simulink model "labFinal_8.slx"  (R2018b)
settings: Solver=FixedStepDiscrete  StartTime=0.0  StopTime=10.0  FixedStep=1  RelTol=1e-3
libraries: hdlsllib x112, simulink_extras x8
(part 2 of 4)

== system labFinal_8.slx/8-Bit_Processor/8-bit Multiply/2^27 ==
  A : Inport
  B : Inport  Port=2
  Cin : Inport  Port=3
  Half_Adder : Subsystem
  Half_Adder1 : Subsystem
  Logical Operator : Logic  Operator=OR  AllPortsSameDT=off  OutDataTypeStr=boolean
  C : Outport
  S : Outport  Port=2
  wires:
  Half_Adder1/1(Sum) -> S/1
  Cin/1 -> Half_Adder1/2(y)
  Logical Operator/1 -> C/1
  Half_Adder1/2(Carry) -> Logical Operator/1
  A/1 -> Half_Adder/1(x)
  B/1 -> Half_Adder/2(y)
  Half_Adder/2(Carry) -> Logical Operator/2
  Half_Adder/1(Sum) -> Half_Adder1/1(x)

== system labFinal_8.slx/8-Bit_Processor/8-bit Multiply/2^28 ==
  A : Inport
  B : Inport  Port=2
  Cin : Inport  Port=3
  Half_Adder : Subsystem
  Half_Adder1 : Subsystem
  Logical Operator : Logic  Operator=OR  AllPortsSameDT=off  OutDataTypeStr=boolean
  C : Outport
  S : Outport  Port=2
  wires:
  Half_Adder1/1(Sum) -> S/1
  Cin/1 -> Half_Adder1/2(y)
  Logical Operator/1 -> C/1
  Half_Adder1/2(Carry) -> Logical Operator/1
  A/1 -> Half_Adder/1(x)
  B/1 -> Half_Adder/2(y)
  Half_Adder/2(Carry) -> Logical Operator/2
  Half_Adder/1(Sum) -> Half_Adder1/1(x)

== system labFinal_8.slx/8-Bit_Processor/8-bit Multiply/2^29 ==
  A : Inport
  B : Inport  Port=2
  Cin : Inport  Port=3
  Half_Adder : Subsystem
  Half_Adder1 : Subsystem
  Logical Operator : Logic  Operator=OR  AllPortsSameDT=off  OutDataTypeStr=boolean
  C : Outport
  S : Outport  Port=2
  wires:
  Half_Adder1/1(Sum) -> S/1
  Cin/1 -> Half_Adder1/2(y)
  Logical Operator/1 -> C/1
  Half_Adder1/2(Carry) -> Logical Operator/1
  A/1 -> Half_Adder/1(x)
  B/1 -> Half_Adder/2(y)
  Half_Adder/2(Carry) -> Logical Operator/2
  Half_Adder/1(Sum) -> Half_Adder1/1(x)

== system labFinal_8.slx/8-Bit_Processor/8-bit Multiply/2^3 ==
  A : Inport
  B : Inport  Port=2
  Cin : Inport  Port=3
  Half_Adder : Subsystem
  Half_Adder1 : Subsystem
  Logical Operator : Logic  Operator=OR  AllPortsSameDT=off  OutDataTypeStr=boolean
  C : Outport
  S : Outport  Port=2
  wires:
  Half_Adder1/1(Sum) -> S/1
  Cin/1 -> Half_Adder1/2(y)
  Logical Operator/1 -> C/1
  Half_Adder1/2(Carry) -> Logical Operator/1
  A/1 -> Half_Adder/1(x)
  B/1 -> Half_Adder/2(y)
  Half_Adder/2(Carry) -> Logical Operator/2
  Half_Adder/1(Sum) -> Half_Adder1/1(x)

== system labFinal_8.slx/8-Bit_Processor/8-bit Multiply/2^30 ==
  A : Inport
  B : Inport  Port=2
  Cin : Inport  Port=3
  Half_Adder : Subsystem
  Half_Adder1 : Subsystem
  Logical Operator : Logic  Operator=OR  AllPortsSameDT=off  OutDataTypeStr=boolean
  C : Outport
  S : Outport  Port=2
  wires:
  Half_Adder1/1(Sum) -> S/1
  Cin/1 -> Half_Adder1/2(y)
  Logical Operator/1 -> C/1
  Half_Adder1/2(Carry) -> Logical Operator/1
  A/1 -> Half_Adder/1(x)
  B/1 -> Half_Adder/2(y)
  Half_Adder/2(Carry) -> Logical Operator/2
  Half_Adder/1(Sum) -> Half_Adder1/1(x)

== system labFinal_8.slx/8-Bit_Processor/8-bit Multiply/2^31 ==
  A : Inport
  B : Inport  Port=2
  Cin : Inport  Port=3
  Half_Adder : Subsystem
  Half_Adder1 : Subsystem
  Logical Operator : Logic  Operator=OR  AllPortsSameDT=off  OutDataTypeStr=boolean
  C : Outport
  S : Outport  Port=2
  wires:
  Half_Adder1/1(Sum) -> S/1
  Cin/1 -> Half_Adder1/2(y)
  Logical Operator/1 -> C/1
  Half_Adder1/2(Carry) -> Logical Operator/1
  A/1 -> Half_Adder/1(x)
  B/1 -> Half_Adder/2(y)
  Half_Adder/2(Carry) -> Logical Operator/2
  Half_Adder/1(Sum) -> Half_Adder1/1(x)

== system labFinal_8.slx/8-Bit_Processor/8-bit Multiply/2^32 ==
  A : Inport
  B : Inport  Port=2
  Cin : Inport  Port=3
  Half_Adder : Subsystem
  Half_Adder1 : Subsystem
  Logical Operator : Logic  Operator=OR  AllPortsSameDT=off  OutDataTypeStr=boolean
  C : Outport
  S : Outport  Port=2
  wires:
  Half_Adder1/1(Sum) -> S/1
  Cin/1 -> Half_Adder1/2(y)
  Logical Operator/1 -> C/1
  Half_Adder1/2(Carry) -> Logical Operator/1
  A/1 -> Half_Adder/1(x)
  B/1 -> Half_Adder/2(y)
  Half_Adder/2(Carry) -> Logical Operator/2
  Half_Adder/1(Sum) -> Half_Adder1/1(x)

== system labFinal_8.slx/8-Bit_Processor/8-bit Multiply/2^33 ==
  A : Inport
  B : Inport  Port=2
  Cin : Inport  Port=3
  Half_Adder : Subsystem
  Half_Adder1 : Subsystem
  Logical Operator : Logic  Operator=OR  AllPortsSameDT=off  OutDataTypeStr=boolean
  C : Outport
  S : Outport  Port=2
  wires:
  Half_Adder1/1(Sum) -> S/1
  Cin/1 -> Half_Adder1/2(y)
  Logical Operator/1 -> C/1
  Half_Adder1/2(Carry) -> Logical Operator/1
  A/1 -> Half_Adder/1(x)
  B/1 -> Half_Adder/2(y)
  Half_Adder/2(Carry) -> Logical Operator/2
  Half_Adder/1(Sum) -> Half_Adder1/1(x)

== system labFinal_8.slx/8-Bit_Processor/8-bit Multiply/2^34 ==
  A : Inport
  B : Inport  Port=2
  Cin : Inport  Port=3
  Half_Adder : Subsystem
  Half_Adder1 : Subsystem
  Logical Operator : Logic  Operator=OR  AllPortsSameDT=off  OutDataTypeStr=boolean
  C : Outport
  S : Outport  Port=2
  wires:
  Half_Adder1/1(Sum) -> S/1
  Cin/1 -> Half_Adder1/2(y)
  Logical Operator/1 -> C/1
  Half_Adder1/2(Carry) -> Logical Operator/1
  A/1 -> Half_Adder/1(x)
  B/1 -> Half_Adder/2(y)
  Half_Adder/2(Carry) -> Logical Operator/2
  Half_Adder/1(Sum) -> Half_Adder1/1(x)

== system labFinal_8.slx/8-Bit_Processor/8-bit Multiply/2^35 ==
  A : Inport
  B : Inport  Port=2
  Cin : Inport  Port=3
  Half_Adder : Subsystem
  Half_Adder1 : Subsystem
  Logical Operator : Logic  Operator=OR  AllPortsSameDT=off  OutDataTypeStr=boolean
  C : Outport
  S : Outport  Port=2
  wires:
  Half_Adder1/1(Sum) -> S/1
  Cin/1 -> Half_Adder1/2(y)
  Logical Operator/1 -> C/1
  Half_Adder1/2(Carry) -> Logical Operator/1
  A/1 -> Half_Adder/1(x)
  B/1 -> Half_Adder/2(y)
  Half_Adder/2(Carry) -> Logical Operator/2
  Half_Adder/1(Sum) -> Half_Adder1/1(x)

== system labFinal_8.slx/8-Bit_Processor/8-bit Multiply/2^36 ==
  A : Inport
  B : Inport  Port=2
  Cin : Inport  Port=3
  Half_Adder : Subsystem
  Half_Adder1 : Subsystem
  Logical Operator : Logic  Operator=OR  AllPortsSameDT=off  OutDataTypeStr=boolean
  C : Outport
  S : Outport  Port=2
  wires:
  Half_Adder1/1(Sum) -> S/1
  Cin/1 -> Half_Adder1/2(y)
  Logical Operator/1 -> C/1
  Half_Adder1/2(Carry) -> Logical Operator/1
  A/1 -> Half_Adder/1(x)
  B/1 -> Half_Adder/2(y)
  Half_Adder/2(Carry) -> Logical Operator/2
  Half_Adder/1(Sum) -> Half_Adder1/1(x)

== system labFinal_8.slx/8-Bit_Processor/8-bit Multiply/2^37 ==
  A : Inport
  B : Inport  Port=2
  Cin : Inport  Port=3
  Half_Adder : Subsystem
  Half_Adder1 : Subsystem
  Logical Operator : Logic  Operator=OR  AllPortsSameDT=off  OutDataTypeStr=boolean
  C : Outport
  S : Outport  Port=2
  wires:
  Half_Adder1/1(Sum) -> S/1
  Cin/1 -> Half_Adder1/2(y)
  Logical Operator/1 -> C/1
  Half_Adder1/2(Carry) -> Logical Operator/1
  A/1 -> Half_Adder/1(x)
  B/1 -> Half_Adder/2(y)
  Half_Adder/2(Carry) -> Logical Operator/2
  Half_Adder/1(Sum) -> Half_Adder1/1(x)

== system labFinal_8.slx/8-Bit_Processor/8-bit Multiply/2^38 ==
  A : Inport
  B : Inport  Port=2
  Cin : Inport  Port=3
  Half_Adder : Subsystem
  Half_Adder1 : Subsystem
  Logical Operator : Logic  Operator=OR  AllPortsSameDT=off  OutDataTypeStr=boolean
  C : Outport
  S : Outport  Port=2
  wires:
  Half_Adder1/1(Sum) -> S/1
  Cin/1 -> Half_Adder1/2(y)
  Logical Operator/1 -> C/1
  Half_Adder1/2(Carry) -> Logical Operator/1
  A/1 -> Half_Adder/1(x)
  B/1 -> Half_Adder/2(y)
  Half_Adder/2(Carry) -> Logical Operator/2
  Half_Adder/1(Sum) -> Half_Adder1/1(x)

== system labFinal_8.slx/8-Bit_Processor/8-bit Multiply/2^39 ==
  A : Inport
  B : Inport  Port=2
  Cin : Inport  Port=3
  Half_Adder : Subsystem
  Half_Adder1 : Subsystem
  Logical Operator : Logic  Operator=OR  AllPortsSameDT=off  OutDataTypeStr=boolean
  C : Outport
  S : Outport  Port=2
  wires:
  Half_Adder1/1(Sum) -> S/1
  Cin/1 -> Half_Adder1/2(y)
  Logical Operator/1 -> C/1
  Half_Adder1/2(Carry) -> Logical Operator/1
  A/1 -> Half_Adder/1(x)
  B/1 -> Half_Adder/2(y)
  Half_Adder/2(Carry) -> Logical Operator/2
  Half_Adder/1(Sum) -> Half_Adder1/1(x)

== system labFinal_8.slx/8-Bit_Processor/8-bit Multiply/2^4 ==
  A : Inport
  B : Inport  Port=2
  Cin : Inport  Port=3
  Half_Adder : Subsystem
  Half_Adder1 : Subsystem
  Logical Operator : Logic  Operator=OR  AllPortsSameDT=off  OutDataTypeStr=boolean
  C : Outport
  S : Outport  Port=2
  wires:
  Half_Adder1/1(Sum) -> S/1
  Cin/1 -> Half_Adder1/2(y)
  Logical Operator/1 -> C/1
  Half_Adder1/2(Carry) -> Logical Operator/1
  A/1 -> Half_Adder/1(x)
  B/1 -> Half_Adder/2(y)
  Half_Adder/2(Carry) -> Logical Operator/2
  Half_Adder/1(Sum) -> Half_Adder1/1(x)

== system labFinal_8.slx/8-Bit_Processor/8-bit Multiply/2^5 ==
  A : Inport
  B : Inport  Port=2
  Cin : Inport  Port=3
  Half_Adder : Subsystem
  Half_Adder1 : Subsystem
  Logical Operator : Logic  Operator=OR  AllPortsSameDT=off  OutDataTypeStr=boolean
  C : Outport
  S : Outport  Port=2
  wires:
  Half_Adder1/1(Sum) -> S/1
  Cin/1 -> Half_Adder1/2(y)
  Logical Operator/1 -> C/1
  Half_Adder1/2(Carry) -> Logical Operator/1
  A/1 -> Half_Adder/1(x)
  B/1 -> Half_Adder/2(y)
  Half_Adder/2(Carry) -> Logical Operator/2
  Half_Adder/1(Sum) -> Half_Adder1/1(x)

== system labFinal_8.slx/8-Bit_Processor/8-bit Multiply/2^6 ==
  A : Inport
  B : Inport  Port=2
  Cin : Inport  Port=3
  Half_Adder : Subsystem
  Half_Adder1 : Subsystem
  Logical Operator : Logic  Operator=OR  AllPortsSameDT=off  OutDataTypeStr=boolean
  C : Outport
  S : Outport  Port=2
  wires:
  Half_Adder1/1(Sum) -> S/1
  Cin/1 -> Half_Adder1/2(y)
  Logical Operator/1 -> C/1
  Half_Adder1/2(Carry) -> Logical Operator/1
  A/1 -> Half_Adder/1(x)
  B/1 -> Half_Adder/2(y)
  Half_Adder/2(Carry) -> Logical Operator/2
  Half_Adder/1(Sum) -> Half_Adder1/1(x)

== system labFinal_8.slx/8-Bit_Processor/8-bit Multiply/2^7 ==
  A : Inport
  B : Inport  Port=2
  Cin : Inport  Port=3
  Half_Adder : Subsystem
  Half_Adder1 : Subsystem
  Logical Operator : Logic  Operator=OR  AllPortsSameDT=off  OutDataTypeStr=boolean
  C : Outport
  S : Outport  Port=2
  wires:
  Half_Adder1/1(Sum) -> S/1
  Cin/1 -> Half_Adder1/2(y)
  Logical Operator/1 -> C/1
  Half_Adder1/2(Carry) -> Logical Operator/1
  A/1 -> Half_Adder/1(x)
  B/1 -> Half_Adder/2(y)
  Half_Adder/2(Carry) -> Logical Operator/2
  Half_Adder/1(Sum) -> Half_Adder1/1(x)

== system labFinal_8.slx/8-Bit_Processor/8-bit Multiply/2^9 ==
  A : Inport
  B : Inport  Port=2
  Cin : Inport  Port=3
  Half_Adder : Subsystem
  Half_Adder1 : Subsystem
  Logical Operator : Logic  Operator=OR  AllPortsSameDT=off  OutDataTypeStr=boolean
  C : Outport
  S : Outport  Port=2
  wires:
  Half_Adder1/1(Sum) -> S/1
  Cin/1 -> Half_Adder1/2(y)
  Logical Operator/1 -> C/1
  Half_Adder1/2(Carry) -> Logical Operator/1
  A/1 -> Half_Adder/1(x)
  B/1 -> Half_Adder/2(y)
  Half_Adder/2(Carry) -> Logical Operator/2
  Half_Adder/1(Sum) -> Half_Adder1/1(x)

== system labFinal_8.slx/8-Bit_Processor/8-bit Multiply/Concat ==
  S 2^0 : Inport
  S 2^1 : Inport  Port=2
  S 2^2 : Inport  Port=3
  S 2^3 : Inport  Port=4
  S 2^4 : Inport  Port=5
  S 2^5 : Inport  Port=6
  S 2^6 : Inport  Port=7
  S 2^7 : Inport  Port=8
  Bit Concat : hdlsllib/Logic and Bit Operations/Bit Concat  numInputs=8
      settings: SourceProductName=HDL Coder  SourceProductBaseCode=HD
  uint11 : Outport
  wires:
  Bit Concat/1 -> uint11/1
  S 2^7/1 -> Bit Concat/1
  S 2^6/1 -> Bit Concat/2
  S 2^5/1 -> Bit Concat/3
  S 2^4/1 -> Bit Concat/4
  S 2^3/1 -> Bit Concat/5
  S 2^2/1 -> Bit Concat/6
  S 2^1/1 -> Bit Concat/7
  S 2^0/1 -> Bit Concat/8

== system labFinal_8.slx/8-Bit_Processor/8-bit Multiply/Half_Adder1 ==
  x : Inport
  y : Inport  Port=2
  Calc Carry : Logic  AllPortsSameDT=off  OutDataTypeStr=boolean
  Calc Sum : Logic  Operator=XOR  AllPortsSameDT=off  OutDataTypeStr=boolean
  C : Outport
  S : Outport  Port=2
  wires:
  Calc Carry/1 -> C/1
  x/1 -> Calc Carry/1, Calc Sum/1
  Calc Sum/1 -> S/1
  y/1 -> Calc Sum/2, Calc Carry/2

== system labFinal_8.slx/8-Bit_Processor/8-bit Multiply/Half_Adder2 ==
  x : Inport
  y : Inport  Port=2
  Calc Carry : Logic  AllPortsSameDT=off  OutDataTypeStr=boolean
  Calc Sum : Logic  Operator=XOR  AllPortsSameDT=off  OutDataTypeStr=boolean
  C : Outport
  S : Outport  Port=2
  wires:
  Calc Carry/1 -> C/1
  x/1 -> Calc Carry/1, Calc Sum/1
  Calc Sum/1 -> S/1
  y/1 -> Calc Sum/2, Calc Carry/2

== system labFinal_8.slx/8-Bit_Processor/8-bit Multiply/Half_Adder3 ==
  x : Inport
  y : Inport  Port=2
  Calc Carry : Logic  AllPortsSameDT=off  OutDataTypeStr=boolean
  Calc Sum : Logic  Operator=XOR  AllPortsSameDT=off  OutDataTypeStr=boolean
  C : Outport
  S : Outport  Port=2
  wires:
  Calc Carry/1 -> C/1
  x/1 -> Calc Carry/1, Calc Sum/1
  Calc Sum/1 -> S/1
  y/1 -> Calc Sum/2, Calc Carry/2

== system labFinal_8.slx/8-Bit_Processor/8-bit Multiply/Half_Adder4 ==
  x : Inport
  y : Inport  Port=2
  Calc Carry : Logic  AllPortsSameDT=off  OutDataTypeStr=boolean
  Calc Sum : Logic  Operator=XOR  AllPortsSameDT=off  OutDataTypeStr=boolean
  C : Outport
  S : Outport  Port=2
  wires:
  Calc Carry/1 -> C/1
  x/1 -> Calc Carry/1, Calc Sum/1
  Calc Sum/1 -> S/1
  y/1 -> Calc Sum/2, Calc Carry/2

== system labFinal_8.slx/8-Bit_Processor/8-bit Multiply/Half_Adder5 ==
  x : Inport
  y : Inport  Port=2
  Calc Carry : Logic  AllPortsSameDT=off  OutDataTypeStr=boolean
  Calc Sum : Logic  Operator=XOR  AllPortsSameDT=off  OutDataTypeStr=boolean
  C : Outport
  S : Outport  Port=2
  wires:
  Calc Carry/1 -> C/1
  x/1 -> Calc Carry/1, Calc Sum/1
  Calc Sum/1 -> S/1
  y/1 -> Calc Sum/2, Calc Carry/2

== system labFinal_8.slx/8-Bit_Processor/8-bit Multiply/Half_Adder6 ==
  x : Inport
  y : Inport  Port=2
  Calc Carry : Logic  AllPortsSameDT=off  OutDataTypeStr=boolean
  Calc Sum : Logic  Operator=XOR  AllPortsSameDT=off  OutDataTypeStr=boolean
  C : Outport
  S : Outport  Port=2
  wires:
  Calc Carry/1 -> C/1
  x/1 -> Calc Carry/1, Calc Sum/1
  Calc Sum/1 -> S/1
  y/1 -> Calc Sum/2, Calc Carry/2

== system labFinal_8.slx/8-Bit_Processor/8-bit Multiply/Half_Adder7 ==
  x : Inport
  y : Inport  Port=2
  Calc Carry : Logic  AllPortsSameDT=off  OutDataTypeStr=boolean
  Calc Sum : Logic  Operator=XOR  AllPortsSameDT=off  OutDataTypeStr=boolean
  C : Outport
  S : Outport  Port=2
  wires:
  Calc Carry/1 -> C/1
  x/1 -> Calc Carry/1, Calc Sum/1
  Calc Sum/1 -> S/1
  y/1 -> Calc Sum/2, Calc Carry/2

== system labFinal_8.slx/8-Bit_Processor/8-bit Multiply/Half_Adder8 ==
  x : Inport
  y : Inport  Port=2
  Calc Carry : Logic  AllPortsSameDT=off  OutDataTypeStr=boolean
  Calc Sum : Logic  Operator=XOR  AllPortsSameDT=off  OutDataTypeStr=boolean
  C : Outport
  S : Outport  Port=2
  wires:
  Calc Carry/1 -> C/1
  x/1 -> Calc Carry/1, Calc Sum/1
  Calc Sum/1 -> S/1
  y/1 -> Calc Sum/2, Calc Carry/2

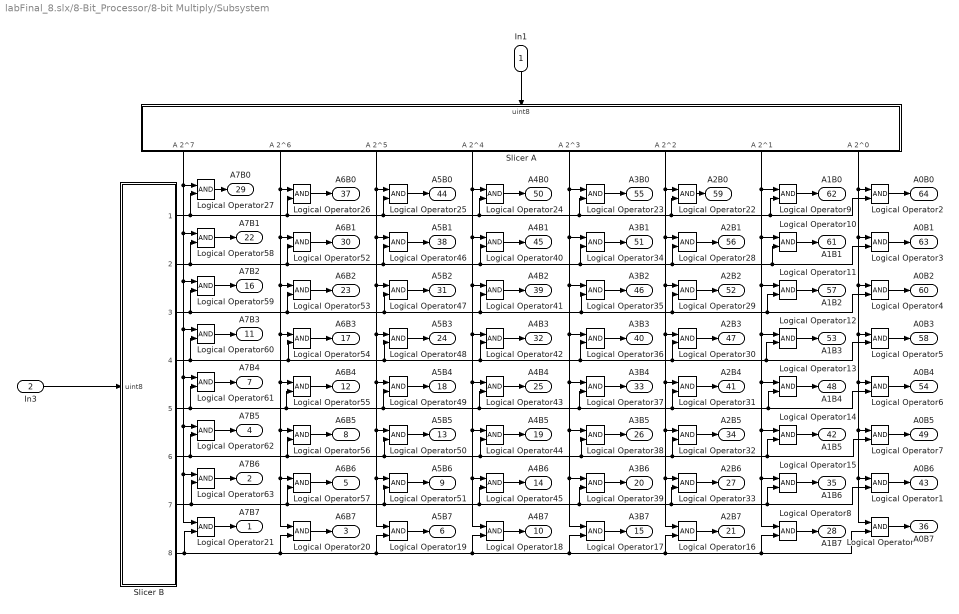
== system labFinal_8.slx/8-Bit_Processor/8-bit Multiply/Subsystem ==
  In1 : Inport
  In3 : Inport  Port=2
  Logical Operator{,1..63} (64 alike) : Logic  AllPortsSameDT=off  OutDataTypeStr=boolean
  Slicer A : Subsystem
  Slicer B : Subsystem
  A7B7 : Outport
  A7B6 : Outport  Port=2
  A6B7 : Outport  Port=3
  A7B5 : Outport  Port=4
  A6B6 : Outport  Port=5
  A5B7 : Outport  Port=6
  A7B4 : Outport  Port=7
  A6B5 : Outport  Port=8
  A5B6 : Outport  Port=9
  A4B7 : Outport  Port=10
  A7B3 : Outport  Port=11
  A6B4 : Outport  Port=12
  A5B5 : Outport  Port=13
  A4B6 : Outport  Port=14
  A3B7 : Outport  Port=15
  A7B2 : Outport  Port=16
  A6B3 : Outport  Port=17
  A5B4 : Outport  Port=18
  A4B5 : Outport  Port=19
  A3B6 : Outport  Port=20
  A2B7 : Outport  Port=21
  A7B1 : Outport  Port=22
  A6B2 : Outport  Port=23
  A5B3 : Outport  Port=24
  A4B4 : Outport  Port=25
  A3B5 : Outport  Port=26
  A2B6 : Outport  Port=27
  A1B7 : Outport  Port=28
  A7B0 : Outport  Port=29
  A6B1 : Outport  Port=30
  A5B2 : Outport  Port=31
  A4B3 : Outport  Port=32
  A3B4 : Outport  Port=33
  A2B5 : Outport  Port=34
  A1B6 : Outport  Port=35
  A0B7 : Outport  Port=36
  A6B0 : Outport  Port=37
  A5B1 : Outport  Port=38
  A4B2 : Outport  Port=39
  A3B3 : Outport  Port=40
  A2B4 : Outport  Port=41
  A1B5 : Outport  Port=42
  A0B6 : Outport  Port=43
  A5B0 : Outport  Port=44
  A4B1 : Outport  Port=45
  A3B2 : Outport  Port=46
  A2B3 : Outport  Port=47
  A1B4 : Outport  Port=48
  A0B5 : Outport  Port=49
  A4B0 : Outport  Port=50
  A3B1 : Outport  Port=51
  A2B2 : Outport  Port=52
  A1B3 : Outport  Port=53
  A0B4 : Outport  Port=54
  A3B0 : Outport  Port=55
  A2B1 : Outport  Port=56
  A1B2 : Outport  Port=57
  A0B3 : Outport  Port=58
  A2B0 : Outport  Port=59
  A0B2 : Outport  Port=60
  A1B1 : Outport  Port=61
  A1B0 : Outport  Port=62
  A0B1 : Outport  Port=63
  A0B0 : Outport  Port=64
  wires:
  Logical Operator48/1 -> A5B3/1
  Logical Operator41/1 -> A4B2/1
  Logical Operator49/1 -> A5B4/1
  Logical Operator23/1 -> A3B0/1
  Logical Operator46/1 -> A5B1/1
  Logical Operator21/1 -> A7B7/1
  Logical Operator26/1 -> A6B0/1
  Logical Operator/1 -> A0B7/1
  Logical Operator43/1 -> A4B4/1
  Logical Operator42/1 -> A4B3/1
  Logical Operator32/1 -> A2B5/1
  Logical Operator5/1 -> A0B3/1
  Logical Operator56/1 -> A6B5/1
  Logical Operator37/1 -> A3B4/1
  Logical Operator50/1 -> A5B5/1
  Logical Operator57/1 -> A6B6/1
  Logical Operator29/1 -> A2B2/1
  Logical Operator39/1 -> A3B6/1
  Slicer B/3(B 2^2) -> Logical Operator59/2, Logical Operator53/2, Logical Operator47/2, Logical Operator41/2, Logical Operator35/2, Logical Operator4/2, Logical Operator11/2, Logical Operator29/2
  Logical Operator1/1 -> A0B6/1
  Logical Operator11/1 -> A1B2/1
  Logical Operator15/1 -> A1B6/1
  Logical Operator47/1 -> A5B2/1
  Slicer B/7(B 2^6) -> Logical Operator63/2, Logical Operator57/2, Logical Operator51/2, Logical Operator45/2, Logical Operator39/2, Logical Operator1/2, Logical Operator15/2, Logical Operator33/2
  Slicer B/5(B 2^4) -> Logical Operator61/2, Logical Operator55/2, Logical Operator49/2, Logical Operator43/2, Logical Operator37/2, Logical Operator6/2, Logical Operator13/2, Logical Operator31/2
  Logical Operator18/1 -> A4B7/1
  Slicer A/3(A 2^5) -> Logical Operator25/1, Logical Operator46/1, Logical Operator47/1, Logical Operator48/1, Logical Operator49/1, Logical Operator50/1, Logical Operator51/1, Logical Operator19/1
  Logical Operator53/1 -> A6B2/1
  Logical Operator55/1 -> A6B4/1
  Logical Operator58/1 -> A7B1/1
  Logical Operator25/1 -> A5B0/1
  Logical Operator59/1 -> A7B2/1
  Logical Operator63/1 -> A7B6/1
  In3/1 -> Slicer B/1(uint8)
  Logical Operator6/1 -> A0B4/1
  Logical Operator4/1 -> A0B2/1
  Slicer B/2(B 2^1) -> Logical Operator58/2, Logical Operator52/2, Logical Operator46/2, Logical Operator40/2, Logical Operator34/2, Logical Operator3/2, Logical Operator10/2, Logical Operator28/2
  Logical Operator12/1 -> A1B3/1
  Logical Operator34/1 -> A3B1/1
  Logical Operator60/1 -> A7B3/1
  Logical Operator31/1 -> A2B4/1
  Logical Operator10/1 -> A1B1/1
  Logical Operator36/1 -> A3B3/1
  Logical Operator35/1 -> A3B2/1
  Logical Operator44/1 -> A4B5/1
  Logical Operator62/1 -> A7B5/1
  Logical Operator51/1 -> A5B6/1
  Slicer A/1(A 2^7) -> Logical Operator27/1, Logical Operator58/1, Logical Operator59/1, Logical Operator60/1, Logical Operator61/1, Logical Operator62/1, Logical Operator63/1, Logical Operator21/1
  Logical Operator24/1 -> A4B0/1
  Logical Operator33/1 -> A2B6/1
  Slicer B/8(B 2^7) -> Logical Operator21/2, Logical Operator20/2, Logical Operator19/2, Logical Operator18/2, Logical Operator17/2, Logical Operator16/2, Logical Operator/2, Logical Operator8/2
  Logical Operator40/1 -> A4B1/1
  Slicer A/6(A 2^2) -> Logical Operator22/1, Logical Operator28/1, Logical Operator29/1, Logical Operator30/1, Logical Operator31/1, Logical Operator32/1, Logical Operator33/1, Logical Operator16/1
  Logical Operator20/1 -> A6B7/1
  Logical Operator3/1 -> A0B1/1
  Logical Operator22/1 -> A2B0/1
  Logical Operator45/1 -> A4B6/1
  Slicer A/4(A 2^4) -> Logical Operator24/1, Logical Operator40/1, Logical Operator41/1, Logical Operator42/1, Logical Operator43/1, Logical Operator44/1, Logical Operator45/1, Logical Operator18/1
  Logical Operator17/1 -> A3B7/1
  Logical Operator30/1 -> A2B3/1
  Logical Operator8/1 -> A1B7/1
  Logical Operator38/1 -> A3B5/1
  Logical Operator13/1 -> A1B4/1
  Logical Operator7/1 -> A0B5/1
  Logical Operator16/1 -> A2B7/1
  Slicer B/1("B 2^0 ") -> Logical Operator26/2, Logical Operator25/2, Logical Operator2/2, Logical Operator9/2, Logical Operator22/2, Logical Operator23/2, Logical Operator24/2, Logical Operator27/2
  Slicer A/8("A 2^0 ") -> Logical Operator2/1, Logical Operator3/1, Logical Operator4/1, Logical Operator5/1, Logical Operator6/1, Logical Operator7/1, Logical Operator1/1, Logical Operator/1
  Logical Operator54/1 -> A6B3/1
  Slicer A/7(A 2^1) -> Logical Operator10/1, Logical Operator11/1, Logical Operator12/1, Logical Operator13/1, Logical Operator14/1, Logical Operator15/1, Logical Operator8/1, Logical Operator9/1
  Logical Operator19/1 -> A5B7/1
  Slicer A/5(A 2^3) -> Logical Operator23/1, Logical Operator34/1, Logical Operator35/1, Logical Operator36/1, Logical Operator37/1, Logical Operator38/1, Logical Operator39/1, Logical Operator17/1
  Logical Operator2/1 -> A0B0/1
  Slicer B/6(B 2^5) -> Logical Operator62/2, Logical Operator56/2, Logical Operator50/2, Logical Operator44/2, Logical Operator7/2, Logical Operator14/2, Logical Operator32/2, Logical Operator38/2
  Logical Operator28/1 -> A2B1/1
  Slicer B/4(B 2^3) -> Logical Operator60/2, Logical Operator54/2, Logical Operator48/2, Logical Operator42/2, Logical Operator36/2, Logical Operator5/2, Logical Operator12/2, Logical Operator30/2
  Logical Operator61/1 -> A7B4/1
  Logical Operator52/1 -> A6B1/1
  In1/1 -> Slicer A/1(uint8)
  Logical Operator14/1 -> A1B5/1
  Logical Operator27/1 -> A7B0/1
  Logical Operator9/1 -> A1B0/1
  Slicer A/2(A 2^6) -> Logical Operator26/1, Logical Operator52/1, Logical Operator53/1, Logical Operator54/1, Logical Operator55/1, Logical Operator56/1, Logical Operator57/1, Logical Operator20/1

== system labFinal_8.slx/8-Bit_Processor/8-bit Register/Concat ==
  S 2^7 : Inport
  S 2^6 : Inport  Port=2
  S 2^5 : Inport  Port=3
  S 2^4 : Inport  Port=4
  S 2^3 : Inport  Port=5
  S 2^2 : Inport  Port=6
  S 2^1 : Inport  Port=7
  S 2^0 : Inport  Port=8
  Bit Concat : hdlsllib/Logic and Bit Operations/Bit Concat  numInputs=8
      settings: SourceProductName=HDL Coder  SourceProductBaseCode=HD
  unsign Int : Outport
  wires:
  Bit Concat/1 -> unsign Int/1
  S 2^3/1 -> Bit Concat/5
  S 2^5/1 -> Bit Concat/3
  S 2^4/1 -> Bit Concat/4
  S 2^0/1 -> Bit Concat/8
  S 2^7/1 -> Bit Concat/1
  S 2^1/1 -> Bit Concat/7
  S 2^6/1 -> Bit Concat/2
  S 2^2/1 -> Bit Concat/6

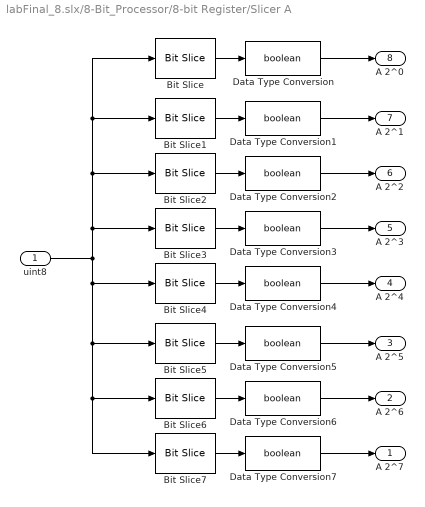
== system labFinal_8.slx/8-Bit_Processor/8-bit Register/Slicer A ==
  uint8 : Inport  OutDataTypeStr=uint8  SampleTime=1
  Bit Slice : hdlsllib/Logic and Bit Operations/Bit Slice  lidx=0  ridx=0
  Bit Slice1 : hdlsllib/Logic and Bit Operations/Bit Slice  lidx=1  ridx=1
  Bit Slice2 : hdlsllib/Logic and Bit Operations/Bit Slice  lidx=2  ridx=2
  Bit Slice3 : hdlsllib/Logic and Bit Operations/Bit Slice  lidx=3  ridx=3
  Bit Slice4 : hdlsllib/Logic and Bit Operations/Bit Slice  lidx=4  ridx=4
  Bit Slice5 : hdlsllib/Logic and Bit Operations/Bit Slice  lidx=5  ridx=5
  Bit Slice6 : hdlsllib/Logic and Bit Operations/Bit Slice  lidx=6  ridx=6
  Bit Slice7 : hdlsllib/Logic and Bit Operations/Bit Slice  lidx=7  ridx=7
  Data Type Conversion{,1..7} (8 alike) : DataTypeConversion  OutDataTypeStr=boolean
  A 2^7 : Outport
  A 2^6 : Outport  Port=2
  A 2^5 : Outport  Port=3
  A 2^4 : Outport  Port=4
  A 2^3 : Outport  Port=5
  A 2^2 : Outport  Port=6
  A 2^1 : Outport  Port=7
  "A 2^0 " : Outport  Port=8
  wires:
  Data Type Conversion/1 -> "A 2^0 "/1
  Data Type Conversion5/1 -> A 2^5/1
  Bit Slice1/1 -> Data Type Conversion1/1
  Bit Slice5/1 -> Data Type Conversion5/1
  Bit Slice7/1 -> Data Type Conversion7/1
  Bit Slice2/1 -> Data Type Conversion2/1
  Bit Slice3/1 -> Data Type Conversion3/1
  Data Type Conversion6/1 -> A 2^6/1
  Bit Slice4/1 -> Data Type Conversion4/1
  uint8/1 -> Bit Slice4/1, Bit Slice5/1, Bit Slice6/1, Bit Slice7/1, Bit Slice3/1, Bit Slice2/1, Bit Slice1/1, Bit Slice/1
  Data Type Conversion1/1 -> A 2^1/1
  Data Type Conversion2/1 -> A 2^2/1
  Bit Slice/1 -> Data Type Conversion/1
  Bit Slice6/1 -> Data Type Conversion6/1
  Data Type Conversion3/1 -> A 2^3/1
  Data Type Conversion4/1 -> A 2^4/1
  Data Type Conversion7/1 -> A 2^7/1

== system labFinal_8.slx/8-Bit_Processor/8-bit Subtractor/2^0 ==
  A : Inport
  B : Inport  Port=2
  Carry In : Inport  Port=3
  Half_Adder : Subsystem
  Half_Adder1 : Subsystem
  Logical Operator : Logic  Operator=OR  AllPortsSameDT=off  OutDataTypeStr=boolean
  Carry : Outport
  Sum : Outport  Port=2
  wires:
  Half_Adder1/1(Sum) -> Sum/1
  Carry In/1 -> Half_Adder1/2(y)
  Logical Operator/1 -> Carry/1
  Half_Adder1/2(Carry) -> Logical Operator/1
  A/1 -> Half_Adder/1(x)
  B/1 -> Half_Adder/2(y)
  Half_Adder/2(Carry) -> Logical Operator/2
  Half_Adder/1(Sum) -> Half_Adder1/1(x)

== system labFinal_8.slx/8-Bit_Processor/8-bit Subtractor/2^1 ==
  A : Inport
  B : Inport  Port=2
  Carry In : Inport  Port=3
  Half_Adder : Subsystem
  Half_Adder1 : Subsystem
  Logical Operator : Logic  Operator=OR  AllPortsSameDT=off  OutDataTypeStr=boolean
  Carry : Outport
  Sum : Outport  Port=2
  wires:
  Half_Adder1/1(Sum) -> Sum/1
  Carry In/1 -> Half_Adder1/2(y)
  Logical Operator/1 -> Carry/1
  Half_Adder1/2(Carry) -> Logical Operator/1
  A/1 -> Half_Adder/1(x)
  B/1 -> Half_Adder/2(y)
  Half_Adder/2(Carry) -> Logical Operator/2
  Half_Adder/1(Sum) -> Half_Adder1/1(x)

== system labFinal_8.slx/8-Bit_Processor/8-bit Subtractor/2^2 ==
  A : Inport
  B : Inport  Port=2
  Carry In : Inport  Port=3
  Half_Adder : Subsystem
  Half_Adder1 : Subsystem
  Logical Operator : Logic  Operator=OR  AllPortsSameDT=off  OutDataTypeStr=boolean
  Carry : Outport
  Sum : Outport  Port=2
  wires:
  Half_Adder1/1(Sum) -> Sum/1
  Carry In/1 -> Half_Adder1/2(y)
  Logical Operator/1 -> Carry/1
  Half_Adder1/2(Carry) -> Logical Operator/1
  A/1 -> Half_Adder/1(x)
  B/1 -> Half_Adder/2(y)
  Half_Adder/2(Carry) -> Logical Operator/2
  Half_Adder/1(Sum) -> Half_Adder1/1(x)

== system labFinal_8.slx/8-Bit_Processor/8-bit Subtractor/2^3 ==
  A : Inport
  B : Inport  Port=2
  Carry In : Inport  Port=3
  Half_Adder : Subsystem
  Half_Adder1 : Subsystem
  Logical Operator : Logic  Operator=OR  AllPortsSameDT=off  OutDataTypeStr=boolean
  Carry : Outport
  Sum : Outport  Port=2
  wires:
  Half_Adder1/1(Sum) -> Sum/1
  Carry In/1 -> Half_Adder1/2(y)
  Logical Operator/1 -> Carry/1
  Half_Adder1/2(Carry) -> Logical Operator/1
  A/1 -> Half_Adder/1(x)
  B/1 -> Half_Adder/2(y)
  Half_Adder/2(Carry) -> Logical Operator/2
  Half_Adder/1(Sum) -> Half_Adder1/1(x)

== system labFinal_8.slx/8-Bit_Processor/8-bit Subtractor/2^4 ==
  A : Inport
  B : Inport  Port=2
  Carry In : Inport  Port=3
  Half_Adder : Subsystem
  Half_Adder1 : Subsystem
  Logical Operator : Logic  Operator=OR  AllPortsSameDT=off  OutDataTypeStr=boolean
  Carry : Outport
  Sum : Outport  Port=2
  wires:
  Half_Adder1/1(Sum) -> Sum/1
  Carry In/1 -> Half_Adder1/2(y)
  Logical Operator/1 -> Carry/1
  Half_Adder1/2(Carry) -> Logical Operator/1
  A/1 -> Half_Adder/1(x)
  B/1 -> Half_Adder/2(y)
  Half_Adder/2(Carry) -> Logical Operator/2
  Half_Adder/1(Sum) -> Half_Adder1/1(x)

== system labFinal_8.slx/8-Bit_Processor/8-bit Subtractor/2^5 ==
  A : Inport
  B : Inport  Port=2
  Carry In : Inport  Port=3
  Half_Adder : Subsystem
  Half_Adder1 : Subsystem
  Logical Operator : Logic  Operator=OR  AllPortsSameDT=off  OutDataTypeStr=boolean
  Carry : Outport
  Sum : Outport  Port=2
  wires:
  Half_Adder1/1(Sum) -> Sum/1
  Carry In/1 -> Half_Adder1/2(y)
  Logical Operator/1 -> Carry/1
  Half_Adder1/2(Carry) -> Logical Operator/1
  A/1 -> Half_Adder/1(x)
  B/1 -> Half_Adder/2(y)
  Half_Adder/2(Carry) -> Logical Operator/2
  Half_Adder/1(Sum) -> Half_Adder1/1(x)

== system labFinal_8.slx/8-Bit_Processor/8-bit Subtractor/2^6 ==
  A : Inport
  B : Inport  Port=2
  Carry In : Inport  Port=3
  Half_Adder : Subsystem
  Half_Adder1 : Subsystem
  Logical Operator : Logic  Operator=OR  AllPortsSameDT=off  OutDataTypeStr=boolean
  Carry : Outport
  Sum : Outport  Port=2
  wires:
  Half_Adder1/1(Sum) -> Sum/1
  Carry In/1 -> Half_Adder1/2(y)
  Logical Operator/1 -> Carry/1
  Half_Adder1/2(Carry) -> Logical Operator/1
  A/1 -> Half_Adder/1(x)
  B/1 -> Half_Adder/2(y)
  Half_Adder/2(Carry) -> Logical Operator/2
  Half_Adder/1(Sum) -> Half_Adder1/1(x)

== system labFinal_8.slx/8-Bit_Processor/8-bit Subtractor/2^7 ==
  A : Inport
  B : Inport  Port=2
  Carry In : Inport  Port=3
  Half_Adder : Subsystem
  Half_Adder1 : Subsystem
  Logical Operator : Logic  Operator=OR  AllPortsSameDT=off  OutDataTypeStr=boolean
  Carry : Outport
  Sum : Outport  Port=2
  wires:
  Half_Adder1/1(Sum) -> Sum/1
  Carry In/1 -> Half_Adder1/2(y)
  Logical Operator/1 -> Carry/1
  Half_Adder1/2(Carry) -> Logical Operator/1
  A/1 -> Half_Adder/1(x)
  B/1 -> Half_Adder/2(y)
  Half_Adder/2(Carry) -> Logical Operator/2
  Half_Adder/1(Sum) -> Half_Adder1/1(x)

== system labFinal_8.slx/8-Bit_Processor/8-bit Subtractor/Concat ==
  S 2^7 : Inport
  S 2^6 : Inport  Port=2
  S 2^5 : Inport  Port=3
  S 2^4 : Inport  Port=4
  S 2^3 : Inport  Port=5
  S 2^2 : Inport  Port=6
  S 2^1 : Inport  Port=7
  S 2^0 : Inport  Port=8
  Bit Concat : hdlsllib/Logic and Bit Operations/Bit Concat  numInputs=8
      settings: SourceProductName=HDL Coder  SourceProductBaseCode=HD
  uint8 : Outport
  wires:
  Bit Concat/1 -> uint8/1
  S 2^3/1 -> Bit Concat/5
  S 2^5/1 -> Bit Concat/3
  S 2^4/1 -> Bit Concat/4
  S 2^0/1 -> Bit Concat/8
  S 2^7/1 -> Bit Concat/1
  S 2^1/1 -> Bit Concat/7
  S 2^6/1 -> Bit Concat/2
  S 2^2/1 -> Bit Concat/6

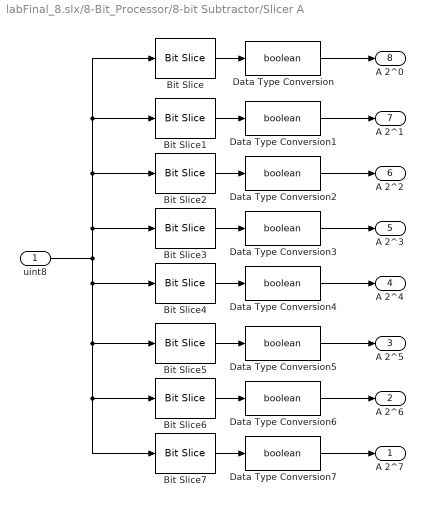
== system labFinal_8.slx/8-Bit_Processor/8-bit Subtractor/Slicer A ==
  uint8 : Inport  OutDataTypeStr=uint8  SampleTime=1
  Bit Slice : hdlsllib/Logic and Bit Operations/Bit Slice  lidx=0  ridx=0
  Bit Slice1 : hdlsllib/Logic and Bit Operations/Bit Slice  lidx=1  ridx=1
  Bit Slice2 : hdlsllib/Logic and Bit Operations/Bit Slice  lidx=2  ridx=2
  Bit Slice3 : hdlsllib/Logic and Bit Operations/Bit Slice  lidx=3  ridx=3
  Bit Slice4 : hdlsllib/Logic and Bit Operations/Bit Slice  lidx=4  ridx=4
  Bit Slice5 : hdlsllib/Logic and Bit Operations/Bit Slice  lidx=5  ridx=5
  Bit Slice6 : hdlsllib/Logic and Bit Operations/Bit Slice  lidx=6  ridx=6
  Bit Slice7 : hdlsllib/Logic and Bit Operations/Bit Slice  lidx=7  ridx=7
  Data Type Conversion{,1..7} (8 alike) : DataTypeConversion  OutDataTypeStr=boolean
  A 2^7 : Outport
  A 2^6 : Outport  Port=2
  A 2^5 : Outport  Port=3
  A 2^4 : Outport  Port=4
  A 2^3 : Outport  Port=5
  A 2^2 : Outport  Port=6
  A 2^1 : Outport  Port=7
  "A 2^0 " : Outport  Port=8
  wires:
  Data Type Conversion/1 -> "A 2^0 "/1
  Data Type Conversion5/1 -> A 2^5/1
  Bit Slice1/1 -> Data Type Conversion1/1
  Bit Slice5/1 -> Data Type Conversion5/1
  Bit Slice7/1 -> Data Type Conversion7/1
  Bit Slice2/1 -> Data Type Conversion2/1
  Bit Slice3/1 -> Data Type Conversion3/1
  Data Type Conversion6/1 -> A 2^6/1
  Bit Slice4/1 -> Data Type Conversion4/1
  uint8/1 -> Bit Slice4/1, Bit Slice5/1, Bit Slice6/1, Bit Slice7/1, Bit Slice3/1, Bit Slice2/1, Bit Slice1/1, Bit Slice/1
  Data Type Conversion1/1 -> A 2^1/1
  Data Type Conversion2/1 -> A 2^2/1
  Bit Slice/1 -> Data Type Conversion/1
  Bit Slice6/1 -> Data Type Conversion6/1
  Data Type Conversion3/1 -> A 2^3/1
  Data Type Conversion4/1 -> A 2^4/1
  Data Type Conversion7/1 -> A 2^7/1

== system labFinal_8.slx/8-Bit_Processor/8-bit Subtractor/Slicer B ==
  uint8 : Inport  OutDataTypeStr=uint8  SampleTime=1
  Bit Slice : hdlsllib/Logic and Bit Operations/Bit Slice  lidx=0  ridx=0
  Bit Slice1 : hdlsllib/Logic and Bit Operations/Bit Slice  lidx=1  ridx=1
  Bit Slice2 : hdlsllib/Logic and Bit Operations/Bit Slice  lidx=2  ridx=2
  Bit Slice3 : hdlsllib/Logic and Bit Operations/Bit Slice  lidx=3  ridx=3
  Bit Slice4 : hdlsllib/Logic and Bit Operations/Bit Slice  lidx=4  ridx=4
  Bit Slice5 : hdlsllib/Logic and Bit Operations/Bit Slice  lidx=5  ridx=5
  Bit Slice6 : hdlsllib/Logic and Bit Operations/Bit Slice  lidx=6  ridx=6
  Bit Slice7 : hdlsllib/Logic and Bit Operations/Bit Slice  lidx=7  ridx=7
  Data Type Conversion{,1..7} (8 alike) : DataTypeConversion  OutDataTypeStr=boolean
  B 2^7 : Outport
  B 2^6 : Outport  Port=2
  B 2^5 : Outport  Port=3
  B 2^4 : Outport  Port=4
  B 2^3 : Outport  Port=5
  B 2^2 : Outport  Port=6
  B 2^1 : Outport  Port=7
  "B 2^0 " : Outport  Port=8
  wires:
  Data Type Conversion/1 -> "B 2^0 "/1
  Data Type Conversion5/1 -> B 2^5/1
  Bit Slice1/1 -> Data Type Conversion1/1
  Bit Slice5/1 -> Data Type Conversion5/1
  Bit Slice7/1 -> Data Type Conversion7/1
  Bit Slice2/1 -> Data Type Conversion2/1
  Bit Slice3/1 -> Data Type Conversion3/1
  Data Type Conversion6/1 -> B 2^6/1
  Bit Slice4/1 -> Data Type Conversion4/1
  uint8/1 -> Bit Slice4/1, Bit Slice5/1, Bit Slice6/1, Bit Slice7/1, Bit Slice3/1, Bit Slice2/1, Bit Slice1/1, Bit Slice/1
  Data Type Conversion1/1 -> B 2^1/1
  Data Type Conversion2/1 -> B 2^2/1
  Bit Slice/1 -> Data Type Conversion/1
  Bit Slice6/1 -> Data Type Conversion6/1
  Data Type Conversion3/1 -> B 2^3/1
  Data Type Conversion4/1 -> B 2^4/1
  Data Type Conversion7/1 -> B 2^7/1

== system labFinal_8.slx/8-Bit_Processor/8-bit_Bitwise_AND/Concat ==
  S 2^7 : Inport
  S 2^6 : Inport  Port=2
  S 2^5 : Inport  Port=3
  S 2^4 : Inport  Port=4
  S 2^3 : Inport  Port=5
  S 2^2 : Inport  Port=6
  S 2^1 : Inport  Port=7
  S 2^0 : Inport  Port=8
  Bit Concat : hdlsllib/Logic and Bit Operations/Bit Concat  numInputs=8
      settings: SourceProductName=HDL Coder  SourceProductBaseCode=HD
  unsign Int : Outport
  wires:
  Bit Concat/1 -> unsign Int/1
  S 2^3/1 -> Bit Concat/5
  S 2^5/1 -> Bit Concat/3
  S 2^4/1 -> Bit Concat/4
  S 2^0/1 -> Bit Concat/8
  S 2^7/1 -> Bit Concat/1
  S 2^1/1 -> Bit Concat/7
  S 2^6/1 -> Bit Concat/2
  S 2^2/1 -> Bit Concat/6

== system labFinal_8.slx/8-Bit_Processor/8-bit_Bitwise_AND/Slicer A ==
  uint8 : Inport  OutDataTypeStr=uint8  SampleTime=1
  Bit Slice : hdlsllib/Logic and Bit Operations/Bit Slice  lidx=0  ridx=0
  Bit Slice1 : hdlsllib/Logic and Bit Operations/Bit Slice  lidx=1  ridx=1
  Bit Slice2 : hdlsllib/Logic and Bit Operations/Bit Slice  lidx=2  ridx=2
  Bit Slice3 : hdlsllib/Logic and Bit Operations/Bit Slice  lidx=3  ridx=3
  Bit Slice4 : hdlsllib/Logic and Bit Operations/Bit Slice  lidx=4  ridx=4
  Bit Slice5 : hdlsllib/Logic and Bit Operations/Bit Slice  lidx=5  ridx=5
  Bit Slice6 : hdlsllib/Logic and Bit Operations/Bit Slice  lidx=6  ridx=6
  Bit Slice7 : hdlsllib/Logic and Bit Operations/Bit Slice  lidx=7  ridx=7
  Data Type Conversion{,1..7} (8 alike) : DataTypeConversion  OutDataTypeStr=boolean
  A 2^7 : Outport
  A 2^6 : Outport  Port=2
  A 2^5 : Outport  Port=3
  A 2^4 : Outport  Port=4
  A 2^3 : Outport  Port=5
  A 2^2 : Outport  Port=6
  A 2^1 : Outport  Port=7
  "A 2^0 " : Outport  Port=8
  wires:
  Data Type Conversion/1 -> "A 2^0 "/1
  Data Type Conversion5/1 -> A 2^5/1
  Bit Slice1/1 -> Data Type Conversion1/1
  Bit Slice5/1 -> Data Type Conversion5/1
  Bit Slice7/1 -> Data Type Conversion7/1
  Bit Slice2/1 -> Data Type Conversion2/1
  Bit Slice3/1 -> Data Type Conversion3/1
  Data Type Conversion6/1 -> A 2^6/1
  Bit Slice4/1 -> Data Type Conversion4/1
  uint8/1 -> Bit Slice4/1, Bit Slice5/1, Bit Slice6/1, Bit Slice7/1, Bit Slice3/1, Bit Slice2/1, Bit Slice1/1, Bit Slice/1
  Data Type Conversion1/1 -> A 2^1/1
  Data Type Conversion2/1 -> A 2^2/1
  Bit Slice/1 -> Data Type Conversion/1
  Bit Slice6/1 -> Data Type Conversion6/1
  Data Type Conversion3/1 -> A 2^3/1
  Data Type Conversion4/1 -> A 2^4/1
  Data Type Conversion7/1 -> A 2^7/1

== system labFinal_8.slx/8-Bit_Processor/8-bit_Bitwise_AND/Slicer B ==
  uint8 : Inport  OutDataTypeStr=uint8  SampleTime=1
  Bit Slice : hdlsllib/Logic and Bit Operations/Bit Slice  lidx=0  ridx=0
  Bit Slice1 : hdlsllib/Logic and Bit Operations/Bit Slice  lidx=1  ridx=1
  Bit Slice2 : hdlsllib/Logic and Bit Operations/Bit Slice  lidx=2  ridx=2
  Bit Slice3 : hdlsllib/Logic and Bit Operations/Bit Slice  lidx=3  ridx=3
  Bit Slice4 : hdlsllib/Logic and Bit Operations/Bit Slice  lidx=4  ridx=4
  Bit Slice5 : hdlsllib/Logic and Bit Operations/Bit Slice  lidx=5  ridx=5
  Bit Slice6 : hdlsllib/Logic and Bit Operations/Bit Slice  lidx=6  ridx=6
  Bit Slice7 : hdlsllib/Logic and Bit Operations/Bit Slice  lidx=7  ridx=7
  Data Type Conversion{,1..7} (8 alike) : DataTypeConversion  OutDataTypeStr=boolean
  B 2^7 : Outport
  B 2^6 : Outport  Port=2
  B 2^5 : Outport  Port=3
  B 2^4 : Outport  Port=4
  B 2^3 : Outport  Port=5
  B 2^2 : Outport  Port=6
  B 2^1 : Outport  Port=7
  "B 2^0 " : Outport  Port=8
  wires:
  Data Type Conversion/1 -> "B 2^0 "/1
  Data Type Conversion5/1 -> B 2^5/1
  Bit Slice1/1 -> Data Type Conversion1/1
  Bit Slice5/1 -> Data Type Conversion5/1
  Bit Slice7/1 -> Data Type Conversion7/1
  Bit Slice2/1 -> Data Type Conversion2/1
  Bit Slice3/1 -> Data Type Conversion3/1
  Data Type Conversion6/1 -> B 2^6/1
  Bit Slice4/1 -> Data Type Conversion4/1
  uint8/1 -> Bit Slice4/1, Bit Slice5/1, Bit Slice6/1, Bit Slice7/1, Bit Slice3/1, Bit Slice2/1, Bit Slice1/1, Bit Slice/1
  Data Type Conversion1/1 -> B 2^1/1
  Data Type Conversion2/1 -> B 2^2/1
  Bit Slice/1 -> Data Type Conversion/1
  Bit Slice6/1 -> Data Type Conversion6/1
  Data Type Conversion3/1 -> B 2^3/1
  Data Type Conversion4/1 -> B 2^4/1
  Data Type Conversion7/1 -> B 2^7/1

== system labFinal_8.slx/8-Bit_Processor/8-bit 4-1 MUX/4-1 MUX 2^1/2-1 MUX1 ==
  S : Inport  OutDataTypeStr=boolean
  I0 : Inport  Port=2  OutDataTypeStr=boolean
  I1 : Inport  Port=3  OutDataTypeStr=boolean
  Logical Operator : Logic  AllPortsSameDT=off  OutDataTypeStr=boolean
  Logical Operator1 : Logic  AllPortsSameDT=off  OutDataTypeStr=boolean
  Logical Operator2 : Logic  Operator=OR  AllPortsSameDT=off  OutDataTypeStr=boolean
  Logical Operator3 : Logic  Operator=NOT  AllPortsSameDT=off  OutDataTypeStr=boolean
  Z : Outport
  wires:
  Logical Operator2/1 -> Z/1
  Logical Operator1/1 -> Logical Operator2/2
  S/1 -> Logical Operator3/1, Logical Operator1/1
  Logical Operator/1 -> Logical Operator2/1
  I0/1 -> Logical Operator/1
  I1/1 -> Logical Operator1/2
  Logical Operator3/1 -> Logical Operator/2

== system labFinal_8.slx/8-Bit_Processor/8-bit 4-1 MUX/4-1 MUX 2^1/2-1 MUX2 ==
  S : Inport  OutDataTypeStr=boolean
  I0 : Inport  Port=2  OutDataTypeStr=boolean
  I1 : Inport  Port=3  OutDataTypeStr=boolean
  Logical Operator : Logic  AllPortsSameDT=off  OutDataTypeStr=boolean
  Logical Operator1 : Logic  AllPortsSameDT=off  OutDataTypeStr=boolean
  Logical Operator2 : Logic  Operator=OR  AllPortsSameDT=off  OutDataTypeStr=boolean
  Logical Operator3 : Logic  Operator=NOT  AllPortsSameDT=off  OutDataTypeStr=boolean
  Z : Outport
  wires:
  Logical Operator2/1 -> Z/1
  Logical Operator1/1 -> Logical Operator2/2
  S/1 -> Logical Operator3/1, Logical Operator1/1
  Logical Operator/1 -> Logical Operator2/1
  I0/1 -> Logical Operator/1
  I1/1 -> Logical Operator1/2
  Logical Operator3/1 -> Logical Operator/2

== system labFinal_8.slx/8-Bit_Processor/8-bit 4-1 MUX/4-1 MUX 2^1/2-1 MUX3 ==
  S : Inport  OutDataTypeStr=boolean
  I0 : Inport  Port=2  OutDataTypeStr=boolean
  I1 : Inport  Port=3  OutDataTypeStr=boolean
  Logical Operator : Logic  AllPortsSameDT=off  OutDataTypeStr=boolean
  Logical Operator1 : Logic  AllPortsSameDT=off  OutDataTypeStr=boolean
  Logical Operator2 : Logic  Operator=OR  AllPortsSameDT=off  OutDataTypeStr=boolean
  Logical Operator3 : Logic  Operator=NOT  AllPortsSameDT=off  OutDataTypeStr=boolean
  Z : Outport
  wires:
  Logical Operator2/1 -> Z/1
  Logical Operator1/1 -> Logical Operator2/2
  S/1 -> Logical Operator3/1, Logical Operator1/1
  Logical Operator/1 -> Logical Operator2/1
  I0/1 -> Logical Operator/1
  I1/1 -> Logical Operator1/2
  Logical Operator3/1 -> Logical Operator/2

== system labFinal_8.slx/8-Bit_Processor/8-bit 4-1 MUX/4-1 MUX 2^2/2-1 MUX1 ==
  S : Inport  OutDataTypeStr=boolean
  I0 : Inport  Port=2  OutDataTypeStr=boolean
  I1 : Inport  Port=3  OutDataTypeStr=boolean
  Logical Operator : Logic  AllPortsSameDT=off  OutDataTypeStr=boolean
  Logical Operator1 : Logic  AllPortsSameDT=off  OutDataTypeStr=boolean
  Logical Operator2 : Logic  Operator=OR  AllPortsSameDT=off  OutDataTypeStr=boolean
  Logical Operator3 : Logic  Operator=NOT  AllPortsSameDT=off  OutDataTypeStr=boolean
  Z : Outport
  wires:
  Logical Operator2/1 -> Z/1
  Logical Operator1/1 -> Logical Operator2/2
  S/1 -> Logical Operator3/1, Logical Operator1/1
  Logical Operator/1 -> Logical Operator2/1
  I0/1 -> Logical Operator/1
  I1/1 -> Logical Operator1/2
  Logical Operator3/1 -> Logical Operator/2

== system labFinal_8.slx/8-Bit_Processor/8-bit 4-1 MUX/4-1 MUX 2^2/2-1 MUX2 ==
  S : Inport  OutDataTypeStr=boolean
  I0 : Inport  Port=2  OutDataTypeStr=boolean
  I1 : Inport  Port=3  OutDataTypeStr=boolean
  Logical Operator : Logic  AllPortsSameDT=off  OutDataTypeStr=boolean
  Logical Operator1 : Logic  AllPortsSameDT=off  OutDataTypeStr=boolean
  Logical Operator2 : Logic  Operator=OR  AllPortsSameDT=off  OutDataTypeStr=boolean
  Logical Operator3 : Logic  Operator=NOT  AllPortsSameDT=off  OutDataTypeStr=boolean
  Z : Outport
  wires:
  Logical Operator2/1 -> Z/1
  Logical Operator1/1 -> Logical Operator2/2
  S/1 -> Logical Operator3/1, Logical Operator1/1
  Logical Operator/1 -> Logical Operator2/1
  I0/1 -> Logical Operator/1
  I1/1 -> Logical Operator1/2
  Logical Operator3/1 -> Logical Operator/2

== system labFinal_8.slx/8-Bit_Processor/8-bit 4-1 MUX/4-1 MUX 2^2/2-1 MUX3 ==
  S : Inport  OutDataTypeStr=boolean
  I0 : Inport  Port=2  OutDataTypeStr=boolean
  I1 : Inport  Port=3  OutDataTypeStr=boolean
  Logical Operator : Logic  AllPortsSameDT=off  OutDataTypeStr=boolean
  Logical Operator1 : Logic  AllPortsSameDT=off  OutDataTypeStr=boolean
  Logical Operator2 : Logic  Operator=OR  AllPortsSameDT=off  OutDataTypeStr=boolean
  Logical Operator3 : Logic  Operator=NOT  AllPortsSameDT=off  OutDataTypeStr=boolean
  Z : Outport
  wires:
  Logical Operator2/1 -> Z/1
  Logical Operator1/1 -> Logical Operator2/2
  S/1 -> Logical Operator3/1, Logical Operator1/1
  Logical Operator/1 -> Logical Operator2/1
  I0/1 -> Logical Operator/1
  I1/1 -> Logical Operator1/2
  Logical Operator3/1 -> Logical Operator/2

== system labFinal_8.slx/8-Bit_Processor/8-bit 4-1 MUX/4-1 MUX 2^3/2-1 MUX1 ==
  S : Inport  OutDataTypeStr=boolean
  I0 : Inport  Port=2  OutDataTypeStr=boolean
  I1 : Inport  Port=3  OutDataTypeStr=boolean
  Logical Operator : Logic  AllPortsSameDT=off  OutDataTypeStr=boolean
  Logical Operator1 : Logic  AllPortsSameDT=off  OutDataTypeStr=boolean
  Logical Operator2 : Logic  Operator=OR  AllPortsSameDT=off  OutDataTypeStr=boolean
  Logical Operator3 : Logic  Operator=NOT  AllPortsSameDT=off  OutDataTypeStr=boolean
  Z : Outport
  wires:
  Logical Operator2/1 -> Z/1
  Logical Operator1/1 -> Logical Operator2/2
  S/1 -> Logical Operator3/1, Logical Operator1/1
  Logical Operator/1 -> Logical Operator2/1
  I0/1 -> Logical Operator/1
  I1/1 -> Logical Operator1/2
  Logical Operator3/1 -> Logical Operator/2

== system labFinal_8.slx/8-Bit_Processor/8-bit 4-1 MUX/4-1 MUX 2^3/2-1 MUX2 ==
  S : Inport  OutDataTypeStr=boolean
  I0 : Inport  Port=2  OutDataTypeStr=boolean
  I1 : Inport  Port=3  OutDataTypeStr=boolean
  Logical Operator : Logic  AllPortsSameDT=off  OutDataTypeStr=boolean
  Logical Operator1 : Logic  AllPortsSameDT=off  OutDataTypeStr=boolean
  Logical Operator2 : Logic  Operator=OR  AllPortsSameDT=off  OutDataTypeStr=boolean
  Logical Operator3 : Logic  Operator=NOT  AllPortsSameDT=off  OutDataTypeStr=boolean
  Z : Outport
  wires:
  Logical Operator2/1 -> Z/1
  Logical Operator1/1 -> Logical Operator2/2
  S/1 -> Logical Operator3/1, Logical Operator1/1
  Logical Operator/1 -> Logical Operator2/1
  I0/1 -> Logical Operator/1
  I1/1 -> Logical Operator1/2
  Logical Operator3/1 -> Logical Operator/2

== system labFinal_8.slx/8-Bit_Processor/8-bit 4-1 MUX/4-1 MUX 2^3/2-1 MUX3 ==
  S : Inport  OutDataTypeStr=boolean
  I0 : Inport  Port=2  OutDataTypeStr=boolean
  I1 : Inport  Port=3  OutDataTypeStr=boolean
  Logical Operator : Logic  AllPortsSameDT=off  OutDataTypeStr=boolean
  Logical Operator1 : Logic  AllPortsSameDT=off  OutDataTypeStr=boolean
  Logical Operator2 : Logic  Operator=OR  AllPortsSameDT=off  OutDataTypeStr=boolean
  Logical Operator3 : Logic  Operator=NOT  AllPortsSameDT=off  OutDataTypeStr=boolean
  Z : Outport
  wires:
  Logical Operator2/1 -> Z/1
  Logical Operator1/1 -> Logical Operator2/2
  S/1 -> Logical Operator3/1, Logical Operator1/1
  Logical Operator/1 -> Logical Operator2/1
  I0/1 -> Logical Operator/1
  I1/1 -> Logical Operator1/2
  Logical Operator3/1 -> Logical Operator/2

== system labFinal_8.slx/8-Bit_Processor/8-bit 4-1 MUX/4-1 MUX 2^4/2-1 MUX1 ==
  S : Inport  OutDataTypeStr=boolean
  I0 : Inport  Port=2  OutDataTypeStr=boolean
  I1 : Inport  Port=3  OutDataTypeStr=boolean
  Logical Operator : Logic  AllPortsSameDT=off  OutDataTypeStr=boolean
  Logical Operator1 : Logic  AllPortsSameDT=off  OutDataTypeStr=boolean
  Logical Operator2 : Logic  Operator=OR  AllPortsSameDT=off  OutDataTypeStr=boolean
  Logical Operator3 : Logic  Operator=NOT  AllPortsSameDT=off  OutDataTypeStr=boolean
  Z : Outport
  wires:
  Logical Operator2/1 -> Z/1
  Logical Operator1/1 -> Logical Operator2/2
  S/1 -> Logical Operator3/1, Logical Operator1/1
  Logical Operator/1 -> Logical Operator2/1
  I0/1 -> Logical Operator/1
  I1/1 -> Logical Operator1/2
  Logical Operator3/1 -> Logical Operator/2

== system labFinal_8.slx/8-Bit_Processor/8-bit 4-1 MUX/4-1 MUX 2^4/2-1 MUX2 ==
  S : Inport  OutDataTypeStr=boolean
  I0 : Inport  Port=2  OutDataTypeStr=boolean
  I1 : Inport  Port=3  OutDataTypeStr=boolean
  Logical Operator : Logic  AllPortsSameDT=off  OutDataTypeStr=boolean
  Logical Operator1 : Logic  AllPortsSameDT=off  OutDataTypeStr=boolean
  Logical Operator2 : Logic  Operator=OR  AllPortsSameDT=off  OutDataTypeStr=boolean
  Logical Operator3 : Logic  Operator=NOT  AllPortsSameDT=off  OutDataTypeStr=boolean
  Z : Outport
  wires:
  Logical Operator2/1 -> Z/1
  Logical Operator1/1 -> Logical Operator2/2
  S/1 -> Logical Operator3/1, Logical Operator1/1
  Logical Operator/1 -> Logical Operator2/1
  I0/1 -> Logical Operator/1
  I1/1 -> Logical Operator1/2
  Logical Operator3/1 -> Logical Operator/2

== system labFinal_8.slx/8-Bit_Processor/8-bit 4-1 MUX/4-1 MUX 2^4/2-1 MUX3 ==
  S : Inport  OutDataTypeStr=boolean
  I0 : Inport  Port=2  OutDataTypeStr=boolean
  I1 : Inport  Port=3  OutDataTypeStr=boolean
  Logical Operator : Logic  AllPortsSameDT=off  OutDataTypeStr=boolean
  Logical Operator1 : Logic  AllPortsSameDT=off  OutDataTypeStr=boolean
  Logical Operator2 : Logic  Operator=OR  AllPortsSameDT=off  OutDataTypeStr=boolean
  Logical Operator3 : Logic  Operator=NOT  AllPortsSameDT=off  OutDataTypeStr=boolean
  Z : Outport
  wires:
  Logical Operator2/1 -> Z/1
  Logical Operator1/1 -> Logical Operator2/2
  S/1 -> Logical Operator3/1, Logical Operator1/1
  Logical Operator/1 -> Logical Operator2/1
  I0/1 -> Logical Operator/1
  I1/1 -> Logical Operator1/2
  Logical Operator3/1 -> Logical Operator/2

== system labFinal_8.slx/8-Bit_Processor/8-bit 4-1 MUX/4-1 MUX 2^5/2-1 MUX1 ==
  S : Inport  OutDataTypeStr=boolean
  I0 : Inport  Port=2  OutDataTypeStr=boolean
  I1 : Inport  Port=3  OutDataTypeStr=boolean
  Logical Operator : Logic  AllPortsSameDT=off  OutDataTypeStr=boolean
  Logical Operator1 : Logic  AllPortsSameDT=off  OutDataTypeStr=boolean
  Logical Operator2 : Logic  Operator=OR  AllPortsSameDT=off  OutDataTypeStr=boolean
  Logical Operator3 : Logic  Operator=NOT  AllPortsSameDT=off  OutDataTypeStr=boolean
  Z : Outport
  wires:
  Logical Operator2/1 -> Z/1
  Logical Operator1/1 -> Logical Operator2/2
  S/1 -> Logical Operator3/1, Logical Operator1/1
  Logical Operator/1 -> Logical Operator2/1
  I0/1 -> Logical Operator/1
  I1/1 -> Logical Operator1/2
  Logical Operator3/1 -> Logical Operator/2

== system labFinal_8.slx/8-Bit_Processor/8-bit 4-1 MUX/4-1 MUX 2^5/2-1 MUX2 ==
  S : Inport  OutDataTypeStr=boolean
  I0 : Inport  Port=2  OutDataTypeStr=boolean
  I1 : Inport  Port=3  OutDataTypeStr=boolean
  Logical Operator : Logic  AllPortsSameDT=off  OutDataTypeStr=boolean
  Logical Operator1 : Logic  AllPortsSameDT=off  OutDataTypeStr=boolean
  Logical Operator2 : Logic  Operator=OR  AllPortsSameDT=off  OutDataTypeStr=boolean
  Logical Operator3 : Logic  Operator=NOT  AllPortsSameDT=off  OutDataTypeStr=boolean
  Z : Outport
  wires:
  Logical Operator2/1 -> Z/1
  Logical Operator1/1 -> Logical Operator2/2
  S/1 -> Logical Operator3/1, Logical Operator1/1
  Logical Operator/1 -> Logical Operator2/1
  I0/1 -> Logical Operator/1
  I1/1 -> Logical Operator1/2
  Logical Operator3/1 -> Logical Operator/2

== system labFinal_8.slx/8-Bit_Processor/8-bit 4-1 MUX/4-1 MUX 2^5/2-1 MUX3 ==
  S : Inport  OutDataTypeStr=boolean
  I0 : Inport  Port=2  OutDataTypeStr=boolean
  I1 : Inport  Port=3  OutDataTypeStr=boolean
  Logical Operator : Logic  AllPortsSameDT=off  OutDataTypeStr=boolean
  Logical Operator1 : Logic  AllPortsSameDT=off  OutDataTypeStr=boolean
  Logical Operator2 : Logic  Operator=OR  AllPortsSameDT=off  OutDataTypeStr=boolean
  Logical Operator3 : Logic  Operator=NOT  AllPortsSameDT=off  OutDataTypeStr=boolean
  Z : Outport
  wires:
  Logical Operator2/1 -> Z/1
  Logical Operator1/1 -> Logical Operator2/2
  S/1 -> Logical Operator3/1, Logical Operator1/1
  Logical Operator/1 -> Logical Operator2/1
  I0/1 -> Logical Operator/1
  I1/1 -> Logical Operator1/2
  Logical Operator3/1 -> Logical Operator/2
